simulink model "puma_model_based"  (R2016b)
settings: Solver=VariableStepAuto  StartTime=0.0  StopTime=10.0  RelTol=1e-3
undefined symbols (not defined in the file): md_d, md_i, md_p, me, mj2, mj3, plan, q_init, tb, X, Y, Z
libraries: sm_lib x18, nesl_utility x10, simulink x6
settings Model: Creator=25097  LastModifiedBy=25097

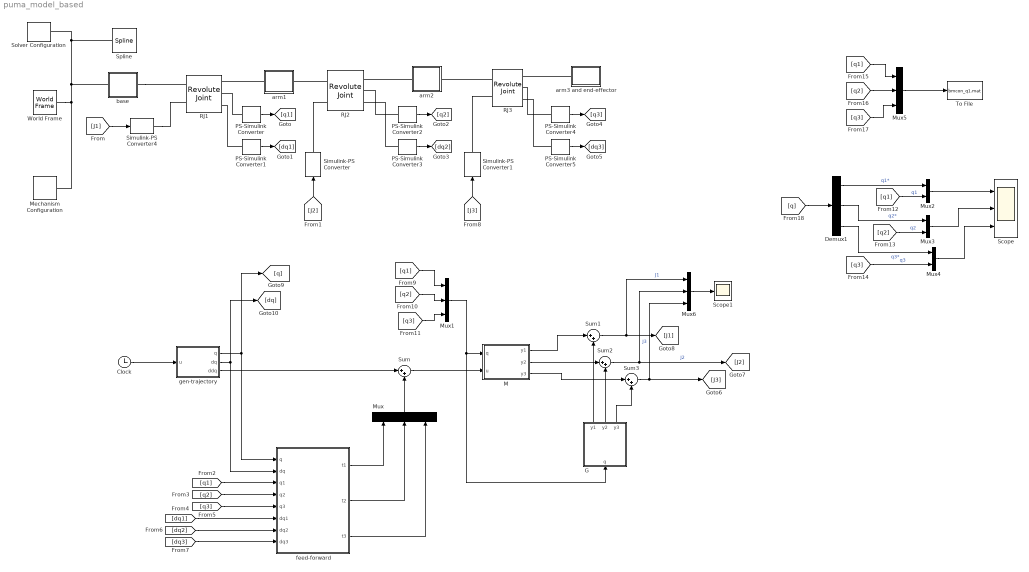
== system puma_model_based ==
  Clock : Clock
  Demux1 : Demux  Outputs=3
  G : MATLAB Function  TreatAsAtomicUnit=on
  M : MATLAB Function  TreatAsAtomicUnit=on
  Mechanism Configuration : sm_lib/Utilities/Mechanism Configuration  UniformGravity=Constant  GravityVector=[0 0 -9.8]  GravityUnits=m/s^2  LinearizationDelta=0.001
  Mux{,1,5..6} (4 alike) : Mux  Inputs=3
  Mux2 : Mux  Inputs=2
  Mux3 : Mux  Inputs=2
  Mux4 : Mux  Inputs=2
  PS-Simulink Converter : nesl_utility/PS-Simulink Converter  PhysicalDomain=network_engine_domain  SubClassName=ps_output  LeftPortType=input  RightPortType=output  PseudoPeriodic=off  Frequencies=[]  Unit=rad  AffineConversion=off
  PS-Simulink Converter1 : nesl_utility/PS-Simulink Converter  PhysicalDomain=network_engine_domain  SubClassName=ps_output  LeftPortType=input  RightPortType=output  PseudoPeriodic=off  Frequencies=[]  Unit=rad/s  AffineConversion=off
  PS-Simulink Converter2 : nesl_utility/PS-Simulink Converter  PhysicalDomain=network_engine_domain  SubClassName=ps_output  LeftPortType=input  RightPortType=output  PseudoPeriodic=off  Frequencies=[]  Unit=rad  AffineConversion=off
  PS-Simulink Converter3 : nesl_utility/PS-Simulink Converter  PhysicalDomain=network_engine_domain  SubClassName=ps_output  LeftPortType=input  RightPortType=output  PseudoPeriodic=off  Frequencies=[]  Unit=rad/s  AffineConversion=off
  PS-Simulink Converter4 : nesl_utility/PS-Simulink Converter  PhysicalDomain=network_engine_domain  SubClassName=ps_output  LeftPortType=input  RightPortType=output  PseudoPeriodic=off  Frequencies=[]  Unit=rad  AffineConversion=off
  PS-Simulink Converter5 : nesl_utility/PS-Simulink Converter  PhysicalDomain=network_engine_domain  SubClassName=ps_output  LeftPortType=input  RightPortType=output  PseudoPeriodic=off  Frequencies=[]  Unit=rad/s  AffineConversion=off
  RJ1 : sm_lib/Joints/Revolute Joint  SenseConstraintForce=off  SenseConstraintForceX=off  SenseConstraintForceY=off  SenseConstraintForceZ=off  SenseConstraintTorque=off  SenseConstraintTorqueX=off  SenseConstraintTorqueY=off  SenseConstraintTorqueZ=off  SenseTotalForce=off  SenseTotalForceX=off  SenseTotalForceY=off  SenseTotalForceZ=off  SenseTotalTorque=off  SenseTotalTorqueX=off  SenseTotalTorqueY=off  SenseTotalTorqueZ=off  CompositeWrenchDir=FollowerOnBase  CompositeWrenchFrame=BaseFrame  EquilibriumPosition=0  EquilibriumPositionUnits=deg  SpringStiffness=0  SpringStiffnessUnits=N*m/deg  DampingCoefficient=0  DampingCoefficientUnits=N*m/(deg/s)  TorqueActuationMode=InputTorque  MotionActuationMode=ComputedMotion  SensePosition=on  SenseVelocity=on  SenseAcceleration=off  SenseTorqueForce=off  PositionTargetSpecify=off  PositionTargetPriority=High  PositionTargetValue=0  PositionTargetValueUnits=deg  VelocityTargetSpecify=off  VelocityTargetPriority=High  VelocityTargetValue=0  VelocityTargetValueUnits=deg/s
  RJ2 : sm_lib/Joints/Revolute Joint  SenseConstraintForce=off  SenseConstraintForceX=off  SenseConstraintForceY=off  SenseConstraintForceZ=off  SenseConstraintTorque=off  SenseConstraintTorqueX=off  SenseConstraintTorqueY=off  SenseConstraintTorqueZ=off  SenseTotalForce=off  SenseTotalForceX=off  SenseTotalForceY=off  SenseTotalForceZ=off  SenseTotalTorque=off  SenseTotalTorqueX=off  SenseTotalTorqueY=off  SenseTotalTorqueZ=off  CompositeWrenchDir=FollowerOnBase  CompositeWrenchFrame=BaseFrame  EquilibriumPosition=0  EquilibriumPositionUnits=deg  SpringStiffness=0  SpringStiffnessUnits=N*m/deg  DampingCoefficient=0  DampingCoefficientUnits=N*m/(deg/s)  TorqueActuationMode=InputTorque  MotionActuationMode=ComputedMotion  SensePosition=on  SenseVelocity=on  SenseAcceleration=off  SenseTorqueForce=off  PositionTargetSpecify=off  PositionTargetPriority=High  PositionTargetValue=0  PositionTargetValueUnits=deg  VelocityTargetSpecify=off  VelocityTargetPriority=High  VelocityTargetValue=0  VelocityTargetValueUnits=deg/s
  RJ3 : sm_lib/Joints/Revolute Joint  SenseConstraintForce=off  SenseConstraintForceX=off  SenseConstraintForceY=off  SenseConstraintForceZ=off  SenseConstraintTorque=off  SenseConstraintTorqueX=off  SenseConstraintTorqueY=off  SenseConstraintTorqueZ=off  SenseTotalForce=off  SenseTotalForceX=off  SenseTotalForceY=off  SenseTotalForceZ=off  SenseTotalTorque=off  SenseTotalTorqueX=off  SenseTotalTorqueY=off  SenseTotalTorqueZ=off  CompositeWrenchDir=FollowerOnBase  CompositeWrenchFrame=BaseFrame  EquilibriumPosition=0  EquilibriumPositionUnits=deg  SpringStiffness=0  SpringStiffnessUnits=N*m/deg  DampingCoefficient=0  DampingCoefficientUnits=N*m/(deg/s)  TorqueActuationMode=InputTorque  MotionActuationMode=ComputedMotion  SensePosition=on  SenseVelocity=on  SenseAcceleration=off  SenseTorqueForce=off  PositionTargetSpecify=off  PositionTargetPriority=High  PositionTargetValue=0  PositionTargetValueUnits=deg  VelocityTargetSpecify=off  VelocityTargetPriority=High  VelocityTargetValue=0  VelocityTargetValueUnits=deg/s
  Scope : Scope  NumInputPorts=3
  Scope1 : Scope
  Simulink-PS Converter : nesl_utility/Simulink-PS Converter  PhysicalDomain=network_engine_domain  SubClassName=ps_input  LeftPortType=input  RightPortType=output  PseudoPeriodic=off  Frequencies=[]  NoiseDistribution=none  NoiseParameters=[]  Unit=1  AffineConversion=off  InputFiltering=off  SimscapeFilterOrder=1  InputFilterTimeConstant=0.001  UdotUserProvided=1
  Simulink-PS Converter1 : nesl_utility/Simulink-PS Converter  PhysicalDomain=network_engine_domain  SubClassName=ps_input  LeftPortType=input  RightPortType=output  PseudoPeriodic=off  Frequencies=[]  NoiseDistribution=none  NoiseParameters=[]  Unit=1  AffineConversion=off  InputFiltering=off  SimscapeFilterOrder=1  InputFilterTimeConstant=0.001  UdotUserProvided=1
  Simulink-PS Converter4 : nesl_utility/Simulink-PS Converter  PhysicalDomain=network_engine_domain  SubClassName=ps_input  LeftPortType=input  RightPortType=output  PseudoPeriodic=off  Frequencies=[]  NoiseDistribution=none  NoiseParameters=[]  Unit=1  AffineConversion=off  InputFiltering=off  SimscapeFilterOrder=1  InputFilterTimeConstant=0.001  UdotUserProvided=1
  Solver Configuration : nesl_utility/Solver Configuration  PhysicalDomain=network_engine_domain  SubClassName=solver  LeftPortType=input  RightPortType=generic  Accelerate=off  Tones=[]  Harmonics=[]  SimulateNoise=off  Profile=off  UseLocalSampling=off  EnableSwitchedLinearOptims=on  FrequencyDomain=off  UseCCode=off  RelTol=0.001  AbsTol=1e-06  MinStep=1e-09  ToWorkspace=off  RevertToSquareIcSolve=off  NumHomotopyIterations=100  PhasorMode=off  PhasorModeNumHarmonics=1  OverrideAbsTol=off  DoDC=off  ResidualTolerance=1e-09  UseLocalSolver=off  LocalSolverChoice=NE_BACKWARD_EULER_ADVANCER  LocalSolverSampleTime=0.001  DoFixedCost=off  MaxNonlinIter=3  MaxModeIter=2  LinearAlgebra=Sparse  DelaysMemoryBudget=1024  AutomaticFiltering=on  FilteringTimeConstant=0.001
  Spline : sm_lib/Curves and Surfaces/Spline  DataPoints=|  DataPointsUnits=m  EndConditionType=Closed  GraphicType=FromGeometry  MarkerShape=Sphere  MarkerSize=30  GraphicVisPropType=AdvancedVisualProperties  GraphicDiffuseColor=[0.4 1.0 0.2]  GraphicSpecularColor=[0.5 0.5 0.5 1.0]  GraphicAmbientColor=[0.15 0.15 0.15 1.0]  GraphicEmissiveColor=[0.0 0.0 0.0 1.0]  GraphicShininess=100  GraphicOpacity=1.0
      | [0.643990476077583	-0.152700000000000	0.943555134969356
      | 0.643990476077583	-0.215073507245328	0.936999415189498
      | 0.643990476077583	-0.274720992922740	0.917618772262136
      | 0.643990476077583	-0.329035575687742	0.886260233281840
      | 0.643990476077583	-0.375643447643218	0.844294316877014
      | 0.643990476077583	-0.412507621135332	0.793555134969356
      | 0.643990476077583	-0.438016954888546	0.736260233281840
      | 0.643990476077583	-0.451056568610482	0.674913673949652
      | 0.643990476077583	-0.451056568610482	0.612196595989060
      | 0.643990476077583	-0.438016954888546	0.550850036656872
      | 0.643990476077583	-0.412507621135332	0.493555134969356
      | 0.643990476077583	-0.375643447643218	0.442815953061699
      | 0.643990476077583	-0.329035575687742	0.400850036656872
      | 0.643990476077583	-0.274720992922740	0.369491497676576
      | 0.643990476077583	-0.215073507245328	0.350110854749214
      | 0.643990476077583	-0.152700000000000	0.343555134969356
      | 0.643990476077583	-0.0903264927546724	0.350110854749214
      | 0.643990476077583	-0.0306790070772601	0.369491497676576
      | 0.643990476077583	0.0236355756877419	0.400850036656872
      | 0.643990476077583	0.0702434476432181	0.442815953061698
      | 0.643990476077583	0.107107621135332	0.493555134969356
      | 0.643990476077583	0.132616954888546	0.550850036656872
      | 0.643990476077583	0.145656568610482	0.612196595989060
      | 0.643990476077583	0.145656568610482	0.674913673949652
      | 0.643990476077583	0.132616954888546	0.736260233281840
      | 0.643990476077583	0.107107621135332	0.793555134969356
      | 0.643990476077583	0.0702434476432184	0.844294316877013
      | 0.643990476077583	0.0236355756877420	0.886260233281840
      | 0.643990476077583	-0.0306790070772597	0.917618772262136
      | 0.643990476077583	-0.0903264927546720	0.936999415189498]
  Sum{,1..3} (4 alike) : Sum  Inputs=|++
  To File : ToFile  Filename=bmcon_q1.mat  MatrixName=bmq1  SaveFormat=Timeseries
  World Frame : sm_lib/Frames and Transforms/World Frame
  arm1 : Subsystem
  arm2 : Subsystem
  arm3 and end-effector : Subsystem
  base : Subsystem
  feed-forward : Subsystem
  gen-trajectory : MATLAB Function  TreatAsAtomicUnit=on
  wires:
  PS-Simulink Converter/1 -> [q1]
  PS-Simulink Converter1/1 -> [dq1]
  PS-Simulink Converter2/1 -> [q2]
  PS-Simulink Converter3/1 -> [dq2]
  PS-Simulink Converter4/1 -> [q3]
  PS-Simulink Converter5/1 -> [dq3]
  [J1] -> Simulink-PS Converter4/1
  [J2] -> Simulink-PS Converter/1
  [J3] -> Simulink-PS Converter1/1
  Clock/1 -> gen-trajectory/1(u)
  gen-trajectory/3(ddq) -> Sum/1
  gen-trajectory/1(q) -> feed-forward/1(q), [q]
  gen-trajectory/2(dq) -> feed-forward/2(dq), [dq]
  [q1] -> feed-forward/3(q1)
  [q2] -> feed-forward/4(q2)
  [q3] -> feed-forward/5(q3)
  [dq1] -> feed-forward/6(dq1)
  [dq2] -> feed-forward/7(dq2)
  [dq3] -> feed-forward/8(dq3)
  feed-forward/1(t1) -> Mux/1
  feed-forward/2(t2) -> Mux/2
  feed-forward/3(t3) -> Mux/3
  Mux/1 -> Sum/2
  Sum/1 -> M/2(u)
  Sum3/1 -> Mux6/3, [J3]  "J3"
  Sum2/1 -> Mux6/2, [J2]  "J2"
  Sum1/1 -> Mux6/1, [J1]  "J1"
  Mux1/1 -> M/1(q), G/1(q)
  [q1] -> Mux1/1
  [q2] -> Mux1/2
  [q3] -> Mux1/3
  [q] -> Demux1/1
  Demux1/1 -> Mux2/1  "q1*"
  [q1] -> Mux2/2  "q1"
  Mux2/1 -> Scope/1
  Demux1/2 -> Mux3/1  "q2*"
  [q2] -> Mux3/2  "q2"
  Mux3/1 -> Scope/2
  Mux4/1 -> Scope/3
  [q3] -> Mux4/2  "q3"
  Demux1/3 -> Mux4/1  "q3*"
  [q1] -> Mux5/1
  [q2] -> Mux5/2
  [q3] -> Mux5/3
  Mux5/1 -> To File/1
  M/1(y1) -> Sum1/1
  G/1(y1) -> Sum1/2
  M/2(y2) -> Sum2/1
  G/2(y2) -> Sum2/2
  G/3(y3) -> Sum3/2
  M/3(y3) -> Sum3/1
  Mux6/1 -> Scope1/1
  connections:
  Mechanism Configuration/RConn1 -- Spline/LConn1 -- Solver Configuration/RConn1 -- base/LConn1 -- World Frame/RConn1
  PS-Simulink Converter1/LConn1 -- RJ1/RConn3
  PS-Simulink Converter5/LConn1 -- RJ3/RConn3
  PS-Simulink Converter2/LConn1 -- RJ2/RConn2
  base/RConn1 -- RJ1/LConn1
  PS-Simulink Converter/LConn1 -- RJ1/RConn2
  PS-Simulink Converter3/LConn1 -- RJ2/RConn3
  RJ2/LConn1 -- arm1/RConn1
  PS-Simulink Converter4/LConn1 -- RJ3/RConn2
  arm1/LConn1 -- RJ1/RConn1
  arm3 and end-effector/LConn1 -- RJ3/RConn1
  RJ3/LConn1 -- arm2/RConn1
  arm2/LConn1 -- RJ2/RConn1
  Simulink-PS Converter/RConn1 -- RJ2/LConn2
  Simulink-PS Converter4/RConn1 -- RJ1/LConn2
  Simulink-PS Converter1/RConn1 -- RJ3/LConn2

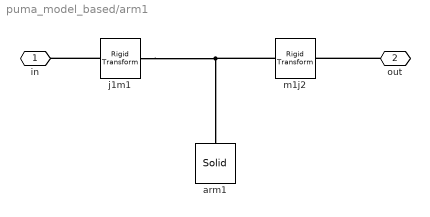
== system puma_model_based/arm1 ==
  arm1 : sm_lib/Body Elements/Solid  InertiaType=Custom  Mass=10  MassUnits=kg  CenterOfMass=[0 0 0.102]  CenterOfMassUnits=m  MomentsOfInertia=[0.05 0.05 0.35]  MomentsOfInertiaUnits=kg*m^2  ProductsOfInertia=[0 0 0]  ProductsOfInertiaUnits=kg*m^2  DensityBased=on  Density=8000  DensityUnits=kg/m^3  DoExposeReferenceFrame=on  SerializedFrames=<Frames/>  GraphicType=FromGeometry  MarkerShape=Sphere  MarkerSize=10  GraphicVisPropType=SimpleVisualProperties  GraphicDiffuseColor=[0.2 0.6 1.0]  GraphicSpecularColor=[0.5 0.5 0.5 1.0]  GraphicAmbientColor=[0.15 0.15 0.15 1.0]  GraphicEmissiveColor=[0.0 0.0 0.0 1.0]  GraphicShininess=75  GraphicOpacity=1.0  GeometryShape=FromFile  RectangleSize=[1 1]  RectangleSizeUnits=m  BrickDimensions=[1 1 1]  BrickDimensionUnits=m  CylinderRadius=1  CylinderRadiusUnits=m  CylinderLength=1  CylinderLengthUnits=m  SphereRadius=1  SphereRadiusUnits=m  EllipsoidRadii=[1 1 1]  EllipsoidRadiiUnits=m  ExtrusionCrossSection=[1 1; -1 1; -1 -1; 1 -1]  ExtrusionCrossSectionUnits=m  ExtrusionLength=1  ExtrusionLengthUnits=m  PolygonNumSides=3  PolygonOuterRadius=1  PolygonOuterRadiusUnits=m  ExtGeomFileType=STL  ExtGeomFileName=C:\Users\25097\Desktop\pmsm\puma560_description-master\meshes\puma_link2.stl  ExtGeomFileUnits=in  RevolutionCrossSection=[1 1; 1 -1; 2 -1; 2 1]  RevolutionCrossSectionUnits=m  RevolutionExtent=Full  RevolutionAngle=180  RevolutionAngleUnits=deg
  j1m1 : sm_lib/Frames and Transforms/Rigid Transform  TranslationMethod=Cartesian  TranslationStandardOffset=0  TranslationLengthUnit=m  TranslationStandardAxis=+Z  TranslationCartesianOffset=[0 0.102 0]  TranslationROffset=0  TranslationROffsetUnits=m  TranslationZOffset=0  TranslationZOffsetUnits=m  TranslationThetaOffset=0  TranslationThetaOffsetUnits=deg  RotationMethod=StandardAxis  RotationAngleUnits=deg  RotationStandardAxis=+X  RotationAngle=90  RotationArbitraryAxis=[0 0 1]  FollAlignAxisA=+X  BaseAlignAxisA=+Y  FollAlignAxisB=+Y  BaseAlignAxisB=+Z  RotationSequenceAxes=FollowerAxes  RotationSequence=XYX  RotationSequenceAngles=[0 0 0]  RotationSequenceAnglesUnits=deg  RotationMatrix=[1 0 0; 0 1 0; 0 0 1]
  m1j2 : sm_lib/Frames and Transforms/Rigid Transform  TranslationMethod=StandardAxis  TranslationStandardOffset=0.30  TranslationLengthUnit=m  TranslationStandardAxis=+Z  TranslationCartesianOffset=[0 0.101 0.6718]  TranslationROffset=0  TranslationROffsetUnits=m  TranslationZOffset=0  TranslationZOffsetUnits=m  TranslationThetaOffset=0  TranslationThetaOffsetUnits=deg  RotationMethod=None  RotationAngleUnits=deg  RotationStandardAxis=+X  RotationAngle=90  RotationArbitraryAxis=[0 0 1]  FollAlignAxisA=+X  BaseAlignAxisA=+Y  FollAlignAxisB=+Y  BaseAlignAxisB=+Z  RotationSequenceAxes=FollowerAxes  RotationSequence=XYX  RotationSequenceAngles=[0 0 0]  RotationSequenceAnglesUnits=deg  RotationMatrix=[1 0 0; 0 1 0; 0 0 1]
  in : PMIOPort  Port=1  Side=Left
  out : PMIOPort  Port=2  Side=Right
  connections:
  j1m1/RConn1 -- m1j2/LConn1 -- arm1/RConn1
  j1m1/LConn1 -- in/RConn1
  out/RConn1 -- m1j2/RConn1

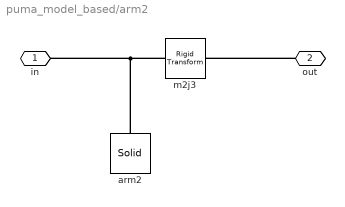
== system puma_model_based/arm2 ==
  arm2 : sm_lib/Body Elements/Solid  InertiaType=Custom  Mass=mj2  MassUnits=kg  CenterOfMass=j2c  CenterOfMassUnits=m  MomentsOfInertia=Ij2  MomentsOfInertiaUnits=kg*m^2  ProductsOfInertia=[0 0 0]  ProductsOfInertiaUnits=kg*m^2  DensityBased=on  Density=8000  DensityUnits=kg/m^3  DoExposeReferenceFrame=on  SerializedFrames=<Frames/>  GraphicType=FromGeometry  MarkerShape=Sphere  MarkerSize=10  GraphicVisPropType=SimpleVisualProperties  GraphicDiffuseColor=[0.0 0.8 0.4]  GraphicSpecularColor=[0.5 0.5 0.5 1.0]  GraphicAmbientColor=[0.15 0.15 0.15 1.0]  GraphicEmissiveColor=[0.0 0.0 0.0 1.0]  GraphicShininess=75  GraphicOpacity=1.0  GeometryShape=FromFile  RectangleSize=[1 1]  RectangleSizeUnits=m  BrickDimensions=[1 1 1]  BrickDimensionUnits=m  CylinderRadius=1  CylinderRadiusUnits=m  CylinderLength=1  CylinderLengthUnits=m  SphereRadius=1  SphereRadiusUnits=m  EllipsoidRadii=[1 1 1]  EllipsoidRadiiUnits=m  ExtrusionCrossSection=[1 1; -1 1; -1 -1; 1 -1]  ExtrusionCrossSectionUnits=m  ExtrusionLength=1  ExtrusionLengthUnits=m  PolygonNumSides=3  PolygonOuterRadius=1  PolygonOuterRadiusUnits=m  ExtGeomFileType=STL  ExtGeomFileName=C:\Users\25097\Desktop\pmsm\puma560_description-master\meshes\puma_link3.stl  ExtGeomFileUnits=in  RevolutionCrossSection=[1 1; 1 -1; 2 -1; 2 1]  RevolutionCrossSectionUnits=m  RevolutionExtent=Full  RevolutionAngle=180  RevolutionAngleUnits=deg
  m2j3 : sm_lib/Frames and Transforms/Rigid Transform  TranslationMethod=Cartesian  TranslationStandardOffset=0.30  TranslationLengthUnit=m  TranslationStandardAxis=+Z  TranslationCartesianOffset=[0.4318 -0.0203 -0.0453]  TranslationROffset=0  TranslationROffsetUnits=m  TranslationZOffset=0  TranslationZOffsetUnits=m  TranslationThetaOffset=0  TranslationThetaOffsetUnits=deg  RotationMethod=StandardAxis  RotationAngleUnits=deg  RotationStandardAxis=+Z  RotationAngle=90  RotationArbitraryAxis=[0 0 1]  FollAlignAxisA=+X  BaseAlignAxisA=+Y  FollAlignAxisB=+Y  BaseAlignAxisB=+Z  RotationSequenceAxes=FollowerAxes  RotationSequence=XYX  RotationSequenceAngles=[0 0 0]  RotationSequenceAnglesUnits=deg  RotationMatrix=[1 0 0; 0 1 0; 0 0 1]
  in : PMIOPort  Port=1  Side=Left
  out : PMIOPort  Port=2  Side=Right
  connections:
  out/RConn1 -- m2j3/RConn1
  m2j3/LConn1 -- arm2/RConn1 -- in/RConn1

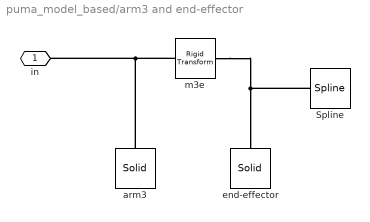
== system puma_model_based/arm3 and end-effector ==
  Spline : sm_lib/Curves and Surfaces/Spline  DataPoints=|  DataPointsUnits=m  EndConditionType=Closed  GraphicType=Marker  MarkerShape=Sphere  MarkerSize=30  GraphicVisPropType=SimpleVisualProperties  GraphicDiffuseColor=[1.0 0.2 0.2]  GraphicSpecularColor=[0.5 0.5 0.5 1.0]  GraphicAmbientColor=[0.15 0.15 0.15 1.0]  GraphicEmissiveColor=[0.0 0.0 0.0 1.0]  GraphicShininess=75  GraphicOpacity=1.0
      | [0.643990476077583	-0.152700000000000	0.943555134969356
      | 0.643990476077583	-0.215073507245328	0.936999415189498
      | 0.643990476077583	-0.274720992922740	0.917618772262136
      | 0.643990476077583	-0.329035575687742	0.886260233281840
      | 0.643990476077583	-0.375643447643218	0.844294316877014
      | 0.643990476077583	-0.412507621135332	0.793555134969356
      | 0.643990476077583	-0.438016954888546	0.736260233281840
      | 0.643990476077583	-0.451056568610482	0.674913673949652
      | 0.643990476077583	-0.451056568610482	0.612196595989060
      | 0.643990476077583	-0.438016954888546	0.550850036656872
      | 0.643990476077583	-0.412507621135332	0.493555134969356
      | 0.643990476077583	-0.375643447643218	0.442815953061699
      | 0.643990476077583	-0.329035575687742	0.400850036656872
      | 0.643990476077583	-0.274720992922740	0.369491497676576
      | 0.643990476077583	-0.215073507245328	0.350110854749214
      | 0.643990476077583	-0.152700000000000	0.343555134969356
      | 0.643990476077583	-0.0903264927546724	0.350110854749214
      | 0.643990476077583	-0.0306790070772601	0.369491497676576
      | 0.643990476077583	0.0236355756877419	0.400850036656872
      | 0.643990476077583	0.0702434476432181	0.442815953061698
      | 0.643990476077583	0.107107621135332	0.493555134969356
      | 0.643990476077583	0.132616954888546	0.550850036656872
      | 0.643990476077583	0.145656568610482	0.612196595989060
      | 0.643990476077583	0.145656568610482	0.674913673949652
      | 0.643990476077583	0.132616954888546	0.736260233281840
      | 0.643990476077583	0.107107621135332	0.793555134969356
      | 0.643990476077583	0.0702434476432184	0.844294316877013
      | 0.643990476077583	0.0236355756877420	0.886260233281840
      | 0.643990476077583	-0.0306790070772597	0.917618772262136
      | 0.643990476077583	-0.0903264927546720	0.936999415189498]
  arm3 : sm_lib/Body Elements/Solid  InertiaType=Custom  Mass=mj3  MassUnits=kg  CenterOfMass=[0.05 0 0]  CenterOfMassUnits=m  MomentsOfInertia=Ij3  MomentsOfInertiaUnits=kg*m^2  ProductsOfInertia=[0 0 0]  ProductsOfInertiaUnits=kg*m^2  DensityBased=on  Density=8000  DensityUnits=kg/m^3  DoExposeReferenceFrame=on  SerializedFrames=<Frames/>  GraphicType=FromGeometry  MarkerShape=Sphere  MarkerSize=10  GraphicVisPropType=SimpleVisualProperties  GraphicDiffuseColor=[1.0 0.8 0.6]  GraphicSpecularColor=[0.5 0.5 0.5 1.0]  GraphicAmbientColor=[0.15 0.15 0.15 1.0]  GraphicEmissiveColor=[0.0 0.0 0.0 1.0]  GraphicShininess=75  GraphicOpacity=1.0  GeometryShape=FromFile  RectangleSize=[1 1]  RectangleSizeUnits=m  BrickDimensions=[1 1 1]  BrickDimensionUnits=m  CylinderRadius=1  CylinderRadiusUnits=m  CylinderLength=1  CylinderLengthUnits=m  SphereRadius=1  SphereRadiusUnits=m  EllipsoidRadii=[1 1 1]  EllipsoidRadiiUnits=m  ExtrusionCrossSection=[1 1; -1 1; -1 -1; 1 -1]  ExtrusionCrossSectionUnits=m  ExtrusionLength=1  ExtrusionLengthUnits=m  PolygonNumSides=3  PolygonOuterRadius=1  PolygonOuterRadiusUnits=m  ExtGeomFileType=STL  ExtGeomFileName=C:\Users\25097\Desktop\pmsm\puma560_description-master\meshes\puma_link4.stl  ExtGeomFileUnits=in  RevolutionCrossSection=[1 1; 1 -1; 2 -1; 2 1]  RevolutionCrossSectionUnits=m  RevolutionExtent=Full  RevolutionAngle=180  RevolutionAngleUnits=deg
  end-effector : sm_lib/Body Elements/Solid  InertiaType=PointMass  Mass=me  MassUnits=kg  CenterOfMass=[0 0 0]  CenterOfMassUnits=m  MomentsOfInertia=[1 1 1]  MomentsOfInertiaUnits=kg*m^2  ProductsOfInertia=[1 1 1]  ProductsOfInertiaUnits=kg*m^2  DensityBased=on  Density=8000  DensityUnits=kg/m^3  DoExposeReferenceFrame=on  SerializedFrames=<Frames/>  GraphicType=FromGeometry  MarkerShape=Sphere  MarkerSize=10  GraphicVisPropType=SimpleVisualProperties  GraphicDiffuseColor=[0.5 0.5 0.5]  GraphicSpecularColor=[0.5 0.5 0.5 1.0]  GraphicAmbientColor=[0.15 0.15 0.15 1.0]  GraphicEmissiveColor=[0.0 0.0 0.0 1.0]  GraphicShininess=75  GraphicOpacity=1.0  GeometryShape=FromFile  RectangleSize=[1 1]  RectangleSizeUnits=m  BrickDimensions=[1 1 1]  BrickDimensionUnits=m  CylinderRadius=1  CylinderRadiusUnits=m  CylinderLength=1  CylinderLengthUnits=m  SphereRadius=1  SphereRadiusUnits=m  EllipsoidRadii=[1 1 1]  EllipsoidRadiiUnits=m  ExtrusionCrossSection=[1 1; -1 1; -1 -1; 1 -1]  ExtrusionCrossSectionUnits=m  ExtrusionLength=1  ExtrusionLengthUnits=m  PolygonNumSides=3  PolygonOuterRadius=1  PolygonOuterRadiusUnits=m  ExtGeomFileType=STL  ExtGeomFileName=C:\Users\25097\Desktop\pmsm\puma560_description-master\meshes\puma_link5.stl  ExtGeomFileUnits=in  RevolutionCrossSection=[1 1; 1 -1; 2 -1; 2 1]  RevolutionCrossSectionUnits=m  RevolutionExtent=Full  RevolutionAngle=180  RevolutionAngleUnits=deg
  m3e : sm_lib/Frames and Transforms/Rigid Transform  TranslationMethod=StandardAxis  TranslationStandardOffset=0.361  TranslationLengthUnit=m  TranslationStandardAxis=+X  TranslationCartesianOffset=[0.4318 -0.0203 -0.0453]  TranslationROffset=0  TranslationROffsetUnits=m  TranslationZOffset=0  TranslationZOffsetUnits=m  TranslationThetaOffset=0  TranslationThetaOffsetUnits=deg  RotationMethod=AlignedAxes  RotationAngleUnits=deg  RotationStandardAxis=+Z  RotationAngle=90  RotationArbitraryAxis=[0 0 1]  FollAlignAxisA=+Z  BaseAlignAxisA=+X  FollAlignAxisB=+X  BaseAlignAxisB=-Z  RotationSequenceAxes=FollowerAxes  RotationSequence=XYX  RotationSequenceAngles=[0 0 0]  RotationSequenceAnglesUnits=deg  RotationMatrix=[1 0 0; 0 1 0; 0 0 1]
  "in " : PMIOPort  Port=1  Side=Left
  connections:
  m3e/RConn1 -- Spline/LConn1 -- end-effector/RConn1
  arm3/RConn1 -- m3e/LConn1 -- "in "/RConn1

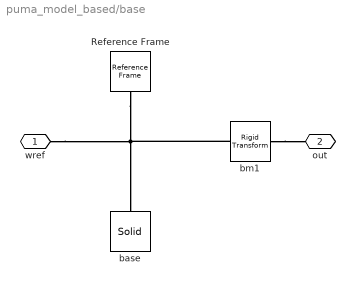
== system puma_model_based/base ==
  Reference Frame : sm_lib/Frames and Transforms/Reference Frame
  base : sm_lib/Body Elements/Solid  InertiaType=Custom  Mass=200  MassUnits=kg  CenterOfMass=[0 0 0]  CenterOfMassUnits=m  MomentsOfInertia=[1 1 1]  MomentsOfInertiaUnits=kg*m^2  ProductsOfInertia=[1 1 1]  ProductsOfInertiaUnits=kg*m^2  DensityBased=on  Density=8000  DensityUnits=kg/m^3  DoExposeReferenceFrame=on  SerializedFrames=<Frames/>  GraphicType=FromGeometry  MarkerShape=Sphere  MarkerSize=10  GraphicVisPropType=SimpleVisualProperties  GraphicDiffuseColor=[0.5 0.5 0.5]  GraphicSpecularColor=[0.5 0.5 0.5 1.0]  GraphicAmbientColor=[0.15 0.15 0.15 1.0]  GraphicEmissiveColor=[0.0 0.0 0.0 1.0]  GraphicShininess=75  GraphicOpacity=1.0  GeometryShape=FromFile  RectangleSize=[1 1]  RectangleSizeUnits=m  BrickDimensions=[1 1 1]  BrickDimensionUnits=m  CylinderRadius=1  CylinderRadiusUnits=m  CylinderLength=1  CylinderLengthUnits=m  SphereRadius=1  SphereRadiusUnits=m  EllipsoidRadii=[1 1 1]  EllipsoidRadiiUnits=m  ExtrusionCrossSection=[1 1; -1 1; -1 -1; 1 -1]  ExtrusionCrossSectionUnits=m  ExtrusionLength=1  ExtrusionLengthUnits=m  PolygonNumSides=3  PolygonOuterRadius=1  PolygonOuterRadiusUnits=m  ExtGeomFileType=STL  ExtGeomFileName=C:\Users\25097\Desktop\pmsm\puma560_description-master\meshes\puma_link1.stl  ExtGeomFileUnits=in  RevolutionCrossSection=[1 1; 1 -1; 2 -1; 2 1]  RevolutionCrossSectionUnits=m  RevolutionExtent=Full  RevolutionAngle=180  RevolutionAngleUnits=deg
  bm1 : sm_lib/Frames and Transforms/Rigid Transform  TranslationMethod=Cartesian  TranslationStandardOffset=0.6718  TranslationLengthUnit=m  TranslationStandardAxis=+Z  TranslationCartesianOffset=[0 0 0.6718]  TranslationROffset=0  TranslationROffsetUnits=m  TranslationZOffset=0  TranslationZOffsetUnits=m  TranslationThetaOffset=0  TranslationThetaOffsetUnits=deg  RotationMethod=None  RotationAngleUnits=deg  RotationStandardAxis=+X  RotationAngle=90  RotationArbitraryAxis=[0 0 1]  FollAlignAxisA=+X  BaseAlignAxisA=+Y  FollAlignAxisB=+Y  BaseAlignAxisB=+Z  RotationSequenceAxes=FollowerAxes  RotationSequence=XYX  RotationSequenceAngles=[0 0 0]  RotationSequenceAnglesUnits=deg  RotationMatrix=[1 0 0; 0 1 0; 0 0 1]
  wref : PMIOPort  Port=1  Side=Left
  out : PMIOPort  Port=2  Side=Right
  connections:
  bm1/RConn1 -- out/RConn1
  bm1/LConn1 -- base/RConn1 -- wref/RConn1 -- Reference Frame/RConn1

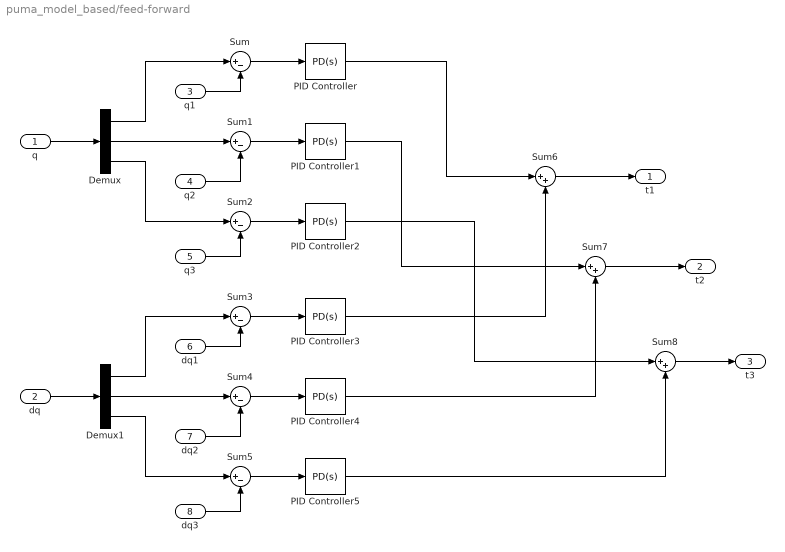
== system puma_model_based/feed-forward ==
  q : Inport
  dq : Inport  Port=2
  q1 : Inport  Port=3
  q2 : Inport  Port=4
  q3 : Inport  Port=5
  dq1 : Inport  Port=6
  dq2 : Inport  Port=7
  dq3 : Inport  Port=8
  Demux : Demux  Outputs=3
  Demux1 : Demux  Outputs=3
  PID Controller{,1..5} (6 alike) : simulink/Continuous/PID Controller  Controller=PD  TimeDomain=Continuous-time  SampleTime=-1  IntegratorMethod=Forward Euler  FilterMethod=Forward Euler  Form=Parallel  UseFilter=on  ControllerParametersSource=internal  P=md_p  I=md_i  D=md_d  N=100  InitialConditionSource=internal  InitialConditionForIntegrator=0  InitialConditionForFilter=0  ExternalReset=none  LimitOutput=off  UpperSaturationLimit=inf  LowerSaturationLimit=-inf  LinearizeAsGain=on  AntiWindupMode=none  Kb=1  TrackingMode=off  Kt=1  PParamMin=[]  PParamMax=[]  IParamMin=[]  IParamMax=[]  DParamMin=[]  DParamMax=[]  NParamMin=[]  NParamMax=[]  KbParamMin=[]  KbParamMax=[]  KtParamMin=[]  KtParamMax=[]  POutMin=[]  POutMax=[]  IOutMin=[]  IOutMax=[]  DOutMin=[]  DOutMax=[]  NOutMin=[]  NOutMax=[]  KbOutMin=[]  KbOutMax=[]  KtOutMin=[]  KtOutMax=[]  IntegratorOutMin=[]  IntegratorOutMax=[]  FilterOutMin=[]  FilterOutMax=[]  SumOutMin=[]  SumOutMax=[]  SumI1OutMin=[]  SumI1OutMax=[]  SumI2OutMin=[]  SumI2OutMax=[]  SumI3OutMin=[]  SumI3OutMax=[]  SumDOutMin=[]  SumDOutMax=[]  SaturationOutMin=[]  SaturationOutMax=[]  IntegratorContinuousStateAttributes=''  IntegratorStateMustResolveToSignalObject=off  IntegratorRTWStateStorageClass=Auto  FilterContinuousStateAttributes=''  FilterStateMustResolveToSignalObject=off  FilterRTWStateStorageClass=Auto  DifferentiatorICPrevScaledInput=0  DifferentiatorOutMin=[]  DifferentiatorOutMax=[]
  Sum{,1..5} (6 alike) : Sum  Inputs=|+-
  Sum6 : Sum  Inputs=|++
  Sum7 : Sum  Inputs=|++
  Sum8 : Sum  Inputs=|++
  t1 : Outport
  t2 : Outport  Port=2
  t3 : Outport  Port=3
  wires:
  q/1 -> Demux/1
  dq/1 -> Demux1/1
  Demux/1 -> Sum/1
  Demux/2 -> Sum1/1
  Demux/3 -> Sum2/1
  q1/1 -> Sum/2
  q2/1 -> Sum1/2
  q3/1 -> Sum2/2
  Sum/1 -> PID Controller/1
  Sum1/1 -> PID Controller1/1
  Sum2/1 -> PID Controller2/1
  Demux1/1 -> Sum3/1
  Demux1/2 -> Sum4/1
  Demux1/3 -> Sum5/1
  dq1/1 -> Sum3/2
  dq2/1 -> Sum4/2
  dq3/1 -> Sum5/2
  Sum3/1 -> PID Controller3/1
  Sum4/1 -> PID Controller4/1
  Sum5/1 -> PID Controller5/1
  PID Controller/1 -> Sum6/1
  PID Controller3/1 -> Sum6/2
  PID Controller1/1 -> Sum7/1
  PID Controller4/1 -> Sum7/2
  PID Controller2/1 -> Sum8/1
  PID Controller5/1 -> Sum8/2
  Sum6/1 -> t1/1
  Sum7/1 -> t2/1
  Sum8/1 -> t3/1

== matlab function puma_model_based/M ==
  data: q input; u input; y1 output; y2 output; y3 output
function [y1,y2,y3] = fcn(q, u)

g = 9.8;
m1 = 10;
m2 = 17.4;
m3 = 4.8;

Iz1 = 0.35;
Ix2 = 0.13;
Iy2 = 0.524;
Iz2 = 0.539;
Ix3 = 0.066;
Iy3 = 0.0125;
Iz3 = 0.086;

p12 = -0.198;
p2c = 0.025;
p3c = 0.05;
p23x = 0.4318;
p23y = -0.0203;
p23z = -0.0453;

q1 = q(1); 
q2 = q(2);
q3 = q(3); 

M1 = [Ix2/2 + Ix3/2 + Iy2/2 + Iy3/2 + Iz1 + m2*p12^2 + m3*p12^2 + (m3*p23x^2)/2 + (m3*p23y^2)/2 + m3*p23z^2 + m2*p2c^2 + (m3*p3c^2)/2 - Ix2*cos(2*q2)/2 + Iy2*cos(2*q2)/2 + Ix3*cos(2*q2 + 2*q3)/2 - Iy3*cos(2*q2 + 2*q3)/2 - 2*m3*p12*p23z - 2*m2*p12*p2c + m3*p23x^2*cos(2*q2)/2 - m3*p23y^2*cos(2*q2)/2 - m3*p3c^2*cos(2*q2 + 2*q3)/2- m3*p23y*p3c*cos(2*q2 + q3) - m3*p23x*p3c*sin(2*q2 + q3)- m3*p23x*p23y*sin(2*q2) + m3*p23y*p3c*cos(q3)- m3*p23x*p3c*sin(q3)
    m3*p12*p3c*cos(q2 + q3)- m3*p23z*p3c*cos(q2 + q3)+ m3*p12*p23y*cos(q2) - m3*p23y*p23z*cos(q2) + m3*p12*p23x*sin(q2) - m3*p23x*p23z*sin(q2) 
    m3*(p12-p23z)*p3c*cos(q2 + q3)
    ];

M2 = [m3*p12*p3c*cos(q2 + q3) - m3*p23z*p3c*cos(q2 + q3) + m3*p12*p23y*cos(q2) - m3*p23y*p23z*cos(q2) + m3*p12*p23x*sin(q2) - m3*p23x*p23z*sin(q2) 
    Iz2 + Iz3 + m3*(p23x^2 + p23y^2) + m3*p3c^2 + 2*m3*p23y*p3c*cos(q3) - 2*m3*p23x*p3c*sin(q3)    
    Iz3 + m3*p3c^2 + m3*p23y*p3c*cos(q3) - m3*p23x*p3c*sin(q3)];

M3 = [m3*p3c*(p12-p23z)*cos(q2 + q3)
    Iz3 + m3*p3c^2 + m3*p3c*(p23y*cos(q3) - p23x*sin(q3))
    Iz3 + m3*p3c^2];

y1 = M1' * u;
y2 = M2' * u;
y3 = M3' * u;

end

== matlab function puma_model_based/gen-trajectory ==
  data: u input; q output; dq output; ddq output; tf parameter; tb parameter; q_init parameter; plan parameter
function [q,dq,ddq] = fcn(u, tf, tb, q_init, plan)
% goto the starting point
if u < tf
    q = 3*q_init/tf^2*u^2 -2*q_init/tf^3*u^3;
    dq = 6*q_init/tf^2*u - 6*q_init/tf^3*u^2;
    ddq = 6*q_init/tf^2 - 12*q_init/tf^3*u;
else if u < tb
    q = q_init;
    dq = zeros(3,1);
    ddq = zeros(3,1);
else
    % start to draw a circle
    tt = 1e-3;
    t = u - tb;
    id = round(t/tt);
    if id == 0
        id = 1;
    end
    if id <= size(plan.q, 2)
        q = plan.q(:,id);
        dq = plan.dq(:,id);
        ddq = plan.ddq(:,id);
    else
        q = plan.q(:,end);
        dq = zeros(3,1);
        ddq = zeros(3,1);
    end
    end

end

== matlab function puma_model_based/G ==
  data: q input; y1 output; y2 output; y3 output
function [y1,y2,y3] = fcn(q)

g = 9.8;
m1 = 10;
m2 = 17.4;
m3 = 4.8;

p12 = -0.198;
p2c = 0.025;
p3c = 0.05;
p23x = 0.4318;
p23y = -0.0203;
p23z = -0.0453;

q1 = q(1); 
q2 = q(2);
q3 = q(3); 

G2 = - g*m3*p3c*sin(q2 + q3) + g*m3*p23x*cos(q2) - g*m3*p23y*sin(q2);
G3 = - m3*p3c*sin(q2 + q3)*g;

y1 = 0;
y2 = G2;
y3 = G3;

end
